simulink model "with_valve_dynamics"  (R2023a)
settings: Solver=ode1  StartTime=0.0  StopTime=0.30  FixedStep=1e-7  MaxStep=1e-6  RelTol=1e-6
InitFcn:
  | %% Parameters
  | 
  | param = struct();
  | 
  | % Volume of chambers
  | param.V1_0 = 1e-3;
  | param.V2_0 = 20e-6;
  | 
  | % Pressure rails
  | param.P_H = 20e6;
  | param.P_M = 10e6;
  | 
  | % Valve things
  | param.max_Avt = 0.5*0.25*pi*(20e-3)^2;
  | param.Cd = 0.6;
  | 
  | % Fluid properties
  | param.beta = 1.8e9;
  | param.rho = 870;
  | 
  | % Electric motor stuff
  | param.Kt = 70.5e-3;
  | param.Ke = 70.5e-3;
  | param.J_elec = 1530e-7;
  | 
  | % Pump things
  | param.J_hyd = 3000e-7;
  | param.hyd_D = 1.6e-6;    % In cc/rev
  | 
  | % Simulation time
  | T = 1;
  | param.on_time = 0;
  | 
  | % Linear Actuator Piston
  | param.Acap = 0.0045;
settings Model: Creator=user  LastModifiedBy=ibrah408

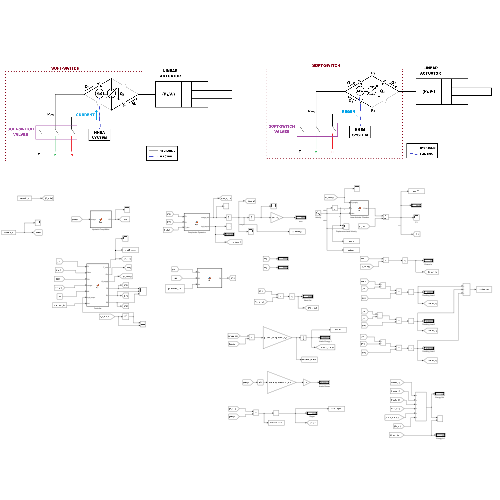
[thumbnail: Simulink's stored preview of the top-level diagram]
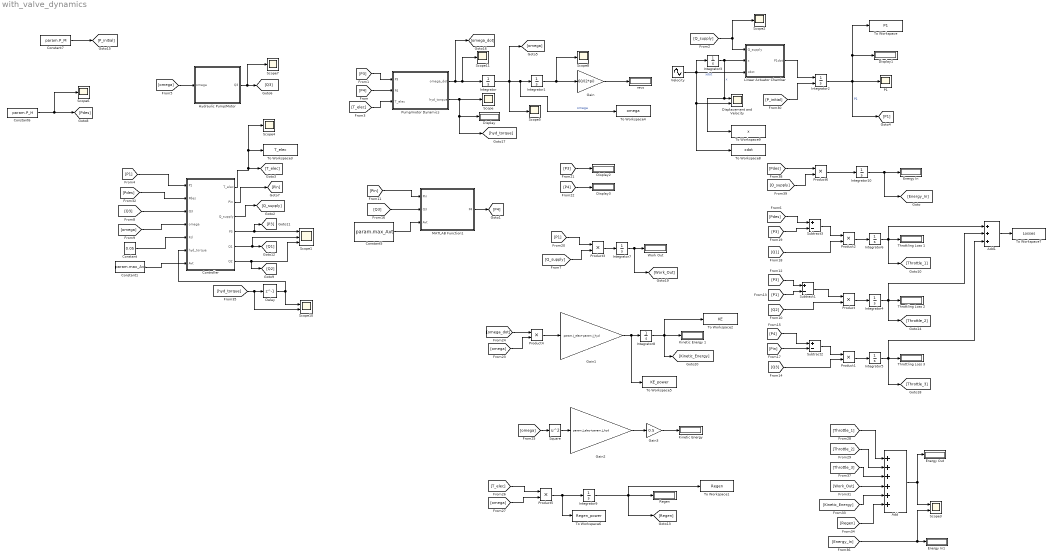
== system with_valve_dynamics ==
  Add : Sum  Inputs=++++++
  Add1 : Sum  Inputs=+++
  Constant : Constant  Value=0.05
  Constant1 : Constant  Value=param.max_Avt
  Constant5 : Constant  Value=param.max_Avt
  Constant6 : Constant  Value=param.P_H
  Constant7 : Constant  Value=param.P_M
  Controller : MATLAB Function  TreatAsAtomicUnit=on
  Delay : Delay  DelayLength=1
  Displacement and Velocity : Scope  NumInputPorts=2
  Display{,1..3} (4 alike) : Display
  Energy In : Display
  Energy In1 : Display
  Energy Out : Display
  Gain : Gain  Gain=60/(2*pi)
  Gain1 : Gain  Gain=param.J_elec+param.J_hyd
  Gain2 : Gain  Gain=param.J_elec+param.J_hyd
  Gain3 : Gain  Gain=0.5
  Hydraulic Pump/Motor : MATLAB Function  TreatAsAtomicUnit=on
  Integrator{,1,3..10} (10 alike) : Integrator
  Integrator2 : Integrator  InitialConditionSource=external  InitialCondition=param.P_M
  Kinetic Energy : Display
  Kinetic Energy 1 : Display
  Linear Actuator Chamber : MATLAB Function  TreatAsAtomicUnit=on
  MATLAB Function1 : MATLAB Function  TreatAsAtomicUnit=on
  P1 : Scope
  Product{,1..6} (7 alike) : Product
  Pump/motor Dynamics : MATLAB Function  TreatAsAtomicUnit=on
  Regen : Display
  Scope{,2,4..8,11} (8 alike) : Scope
  Scope1 : Scope  NumInputPorts=3
  Scope10 : Scope  NumInputPorts=2
  Scope3 : Scope  NumInputPorts=2
  Square : Math  Operator=square
  Subtract1 : Sum  Inputs=+-
  Subtract2 : Sum  Inputs=+-
  Subtract3 : Sum  Inputs=+-
  Throttling Loss 1 : Display
  Throttling Loss 2 : Display
  Throttling Loss 3 : Display
  To Workspace : ToWorkspace  VariableName=P1  SaveFormat=Timeseries  SampleTime=-1
  To Workspace1 : ToWorkspace  VariableName=Regen  SaveFormat=Timeseries  SampleTime=-1
  To Workspace2 : ToWorkspace  VariableName=KE  SaveFormat=Timeseries  SampleTime=-1
  To Workspace3 : ToWorkspace  VariableName=T_elec  SaveFormat=Timeseries  SampleTime=-1
  To Workspace4 : ToWorkspace  VariableName=omega  SaveFormat=Timeseries  SampleTime=-1
  To Workspace5 : ToWorkspace  VariableName=KE_power  SaveFormat=Timeseries  SampleTime=-1
  To Workspace6 : ToWorkspace  VariableName=Regen_power  SaveFormat=Timeseries  SampleTime=-1
  To Workspace7 : ToWorkspace  VariableName=Losses  SaveFormat=Timeseries  SampleTime=-1
  To Workspace8 : ToWorkspace  VariableName=xdot  SaveFormat=Timeseries  SampleTime=-1
  To Workspace9 : ToWorkspace  VariableName=x  SaveFormat=Timeseries  SampleTime=-1
  Velocity : Sin  Amplitude=2e-2  Frequency=2*(2*pi)/0.3  Phase=-pi/2  SampleTime=0
  Work Out : Display
  revs : Display
  wires:
  Pump/motor Dynamics/1(omega_dot) -> [omega_dot], Scope11/1, Integrator/1
  Integrator/1 -> Scope5/1, [omega], To Workspace4/1, Integrator1/1  "omega"
  Integrator1/1 -> Scope8/1, Gain/1
  Gain/1 -> revs/1
  Linear Actuator Chamber/1(P1dot) -> Integrator2/1
  Integrator2/1 -> [P1], To Workspace/1, Display1/1, P1/1  "P1"
  Constant/1 -> Controller/5(Kd)
  [P4] -> Pump/motor Dynamics/2(P4)
  [P3] -> Pump/motor Dynamics/1(P3)
  Controller/3(Q_supply) -> [Q_supply]
  [Q_supply] -> Linear Actuator Chamber/1(Q_supply), Scope2/1
  Controller/1(T_elec) -> Scope4/1, To Workspace3/1, [T_elec]
  [T_elec] -> Pump/motor Dynamics/3(T_elec)
  [P1] -> Controller/1(P1)
  [Pdes] -> Controller/2(Pdes)
  [omega] -> Hydraulic Pump/Motor/1(omega)
  Hydraulic Pump/Motor/1(Q3) -> Scope7/1, [Q3]
  [omega] -> Controller/4(omega)
  Controller/2(Pin) -> [Pin]
  Pump/motor Dynamics/2(hyd_torque) -> [hyd_torque], Display/1, Scope/1
  [P_initial] -> Integrator2/2
  Constant7/1 -> [P_initial]
  Constant6/1 -> [Pdes], Scope6/1
  [hyd_torque] -> Scope10/2, Delay/1
  [Q3] -> Controller/3(Q3)
  [Pin] -> MATLAB Function1/1(Pin)
  MATLAB Function1/1(P4) -> [P4]
  [Q3] -> MATLAB Function1/2(Q3)
  Constant5/1 -> MATLAB Function1/3(Avt)
  Controller/4(P3) -> [P3], Scope1/1
  Constant1/1 -> Controller/7(Avt)
  Velocity/1 -> Displacement and Velocity/2, To Workspace8/1, Linear Actuator Chamber/3(xdot), Integrator3/1  "xdot"
  Integrator3/1 -> Linear Actuator Chamber/2(x), To Workspace9/1, Displacement and Velocity/1  "x"
  [P3] -> Subtract1/1
  [P1] -> Subtract1/2
  [Q2] -> Product/2
  Subtract1/1 -> Product/1
  Product/1 -> Integrator4/1
  Integrator4/1 -> Add1/2, [Throttle_2], Throttling Loss 2/1
  Subtract2/1 -> Product1/1
  [Q3] -> Product1/2
  Product1/1 -> Integrator5/1
  Integrator5/1 -> Add1/3, [Throttle_3], Throttling Loss 3/1
  Controller/6(Q2) -> Scope1/3, [Q2]
  Subtract3/1 -> Product2/1
  [Q1] -> Product2/2
  Product2/1 -> Integrator6/1
  Integrator6/1 -> [Throttle_1], Add1/1, Throttling Loss 1/1
  [P1] -> Product3/1
  [Q_supply] -> Product3/2
  Product3/1 -> Integrator7/1
  Integrator7/1 -> [Work_Out], Work Out/1
  [P4] -> Display3/1
  [P3] -> Display2/1
  [omega_dot] -> Product4/1
  [omega] -> Product4/2
  Product4/1 -> Gain1/1
  Gain1/1 -> To Workspace5/1, Integrator8/1
  Integrator8/1 -> [Kinetic_Energy], To Workspace2/1, Kinetic Energy 1/1
  Gain2/1 -> Gain3/1
  [omega] -> Square/1
  Square/1 -> Gain2/1
  Gain3/1 -> Kinetic Energy/1
  [Pin] -> Subtract2/2
  [P4] -> Subtract2/1
  Controller/5(Q1) -> Scope1/2, [Q1]
  [Pdes] -> Subtract3/1
  [P3] -> Subtract3/2
  [omega] -> Product5/2
  Integrator9/1 -> To Workspace1/1, [Regen], Regen/1
  Product5/1 -> To Workspace6/1, Integrator9/1
  [T_elec] -> Product5/1
  [Energy_In] -> Energy In1/1, Scope3/2
  Add/1 -> Energy Out/1, Scope3/1
  [Throttle_2] -> Add/2
  [Throttle_1] -> Add/1
  [Throttle_3] -> Add/3
  [Work_Out] -> Add/4
  [Kinetic_Energy] -> Add/5
  [Regen] -> Add/6
  Add1/1 -> To Workspace7/1
  [Pdes] -> Product6/1
  [Q_supply] -> Product6/2
  Product6/1 -> Integrator10/1
  Integrator10/1 -> [Energy_In], Energy In/1
  Delay/1 -> Controller/6(hyd_torque), Scope10/1

== matlab function with_valve_dynamics/Pump//motor Dynamics ==
  data: omega_dot output; P3 input; P4 input; param parameter; T_elec input; hyd_torque output
function [omega_dot, hyd_torque] = fcn(P3, P4, param, T_elec)

hyd_torque = (param.hyd_D/(2*pi))*(P3-P4);
omega_dot = (1/(param.J_elec+param.J_hyd))*(hyd_torque - T_elec);

== matlab function with_valve_dynamics/Hydraulic Pump//Motor ==
  data: Q3 output; omega input; param parameter
function Q3   = fcn(omega, param)

Q3 = (param.hyd_D/(2*pi))*omega;

== matlab function with_valve_dynamics/Linear Actuator Chamber ==
  data: P1dot output; Q_supply input; param parameter; x input; xdot input
function P1dot = fcn(Q_supply, param, x, xdot)

P1dot = (param.beta/(param.V1_0+param.Acap*x))*(Q_supply-param.Acap*xdot);

== matlab function with_valve_dynamics/Controller ==
  data: P1 input; Pdes input; Q3 input; omega input; Kd input; param parameter; T_elec output; Pin output; Q_supply output; hyd_torque input; P3 output; Q1 output; Avt input; Q2 output
function [T_elec, Pin, Q_supply, P3, Q1, Q2] = fcn(P1, Pdes, Q3, omega, Kd, param, hyd_torque, Avt)

k = param.Cd*Avt*sqrt(2/param.rho);

if abs(P1-Pdes)<1e4 

    % Phase 2

    sigma = sqrt(abs(2*Pdes*k^2-2*P1*k^2-Q3^2))*sign(2*Pdes*k^2-2*P1*k^2-Q3^2);
    P3 = P1/2 + Pdes/2 - (Q3*sigma)/(2*k^2);
    Q1 = k*sqrt(abs(Pdes-P3))*sign(Pdes-P3);

    Q2 = Q1 - Q3;
    % Q2 = 0;

    if omega < 1
        T_elec = Kd*omega;
        Pin = Pdes;
        Q_supply = Q2;
    else
        T_elec = 30;
        Pin = Pdes;
        Q_supply = Q2;
    end
else

    % Phase 1

    P3 = Pdes - (Q3/k)^2;

    Q1 = Q3;

    Q2 = Q1-Q3;

    if omega >= 300
        T_elec = hyd_torque;
        Pin = P1;
        Q_supply = Q3;
    else
        T_elec = -30;
        Pin = P1;
        Q_supply = Q3;
    end
end

== matlab function with_valve_dynamics/MATLAB Function1 ==
  data: Pin input; P4 output; Q3 input; param parameter; Avt input
function P4 = fcn(Pin, Q3, param, Avt)

k = param.Cd*Avt*sqrt(2/param.rho);
P4 = Pin + (Q3/k)^2;
